simulink model "airgk"  (Simulink 3.00)
settings: Solver=ode45  StartTime=0  StopTime=Inf  RelTol=1e-3
libraries: simulink3 x21, airlib x1
(part 1 of 2)
settings Model: SaveTime=off  SaveOutput=off  RTWOptions="-aEnforceIntegerDowncast=1 -aFoldNonRolledExpr=1 -aInlineInvariantSignals=1 -aInlineParameters=0 -aLocalBlockOutputs=1 -aRollThreshold=5 -aZeroInternalMemoryAtStartup=1 -aZeroExternalMemoryAtStartup=1 -aInitFltsAndDblsToZero=1 -aGenerateReport=0 -aGenCodeOnly=0 -aRTWVerbose=1 -aIncludeHyperlinkInReport=0 -aLaunchReport=0 -aForceParamTrailComments=0 -aGenerateComments=1 -aIgnoreCustomStorageClasses=1 -aIncHierarchyInIds=0 -aMaxRTWIdLen=31 -aShowEliminatedStatements=0 -aPrefixModelToSubsysFcnNames=1 -aIncDataTypeInIds=0 -aInsertBlockDesc=0 -aSimulinkBlockComments=1 -aInlinedPrmAccess=\"Literals\"  -aSuppressErrorStatus=0 -aModelReferenceCompliant=1 -aSupportNonInlinedSFcns=1 -aSupportContinuousTime=1 -aSupportComplex=1 -aSupportNonFinite=1 -aSupportAbsoluteTime=1 -aTargetFcnLib=\"ansi_tfl_tmw.mat\" -aMultiInstanceERTCode=0 -aLogVarNameModifier=\"rt_\" -aIsPILTarget=0 -aCombineOutputUpdateFcns=0 -aGenerateASAP2=0 -aGenerateSampleERTMain=0 -aGenerateFullHeader=1 -aUtilityFuncGeneration=\"Auto\" -aIncludeFileDelimiter=\"Auto\" -aIncludeMdlTerminateFcn=1 -aPurelyIntegerCode=0 -aERTCustomFileBanners=0 -aRTWCAPIStates=0 -aRTWCAPIParams=0 -aRTWCAPISignals=0 -aMatFileLogging=1 -aGenFloatMathFcnCalls=\"ANSI_C\" -aExtModeMexFile=\"ext_comm\" -aExtModeTransport=0 -aExtModeStaticAllocSize=1000000 -aExtModeTesting=0 -aExtModeStaticAlloc=0 -aExtMode=0"  ExtModeTrigMode=normal  ExtModeArmWhenConnect=on  LastModifiedBy=gcampa

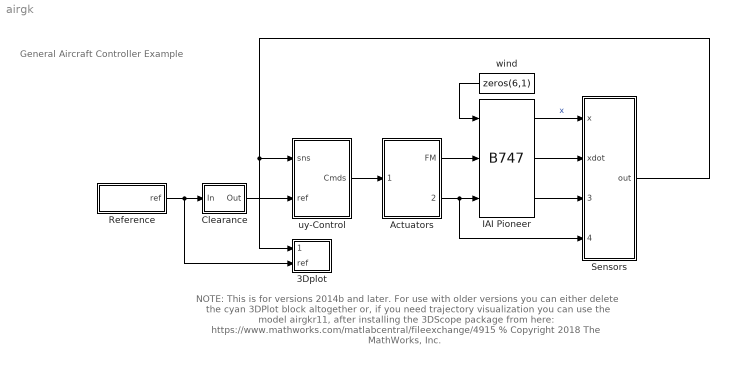
== system airgk ==
  note: General Aircraft
      | Controller Example
  note: NOTE: This is for versions 2014b and later. For use with older versions you can either delete the cyan 3DPlot block altogether or,
      | if you need trajectory visualization you can use the model airgkr11, after installing the 3DScope package from here:
      | https://www.mathworks.com/matlabcentral/fileexchange/4915                                             % Copyright 2018 The MathWorks, Inc.
  " IAI Pioneer " : airlib/B747  GM1="[0.5486  5.1511  2.8261   47.2259  90.9483  111.4754   0  -6.6462  0   190.512]"  CD_wind="[0.060  0.430  0  0.0180  0]"  CL_wind="[0.385  4.78  8.05  0.401  0]"  Cm_body="[0.194  -2.12   -36.6   -1.76    0]"  CY_body="[0   -0.819    0     0    0.191    0]"  Cl_body="[0   -0.023   -0.450   0.265   -0.161  -0.00229]"  Cn_body="[0    0.109  -0.110  -0.200    0.0200  -0.0917]"  x0="[60 -0.0293682 0   0 0 0   0 -0.0293682 0   0 0 60]"
  3Dplot : Subsystem
  Actuators : Subsystem
  Clearance : Subsystem  mask(Reference Position){FC=0, LC=0, HC=0}
      mask prompts: FC "Forward Clearance"; LC "Lateral Clearance"; HC "Altitude Clearance"
      mask help:
      | The input vector contains a position, velocity
      |   and two aditional signals. The output position
      |   is translated respect to the input of the quantities
      |   [FC, LC, HC] respectively behind, on the right
      |   and above the velocity vector direction.
      mask Help:
      | The input vector contains a position, velocity
      |   and two aditional signals. The output position
      |   is translated respect to the input of the quantities
      |   [FC, LC, HC] respectively behind, on the right
      |   and above the velocity vector direction.
  Reference : Subsystem  mask(Reference Path Generation){Px=[0          2000          2000             0             0             0], Py=[0             0          2000          2000          1000             0], Ph=[60           100            60           500            60            60], Pt=[0   33.3400   66.6800  100.8105  119.0191  135.6858], T=0.05}
      mask prompts: Px "X Positions"; Py "Y Positions"; Ph "H Positions"; Pt "Time"; T "Sample Time"
      mask help: This block generates a 3D trajectory. The output is a vector containing the position and velocity of a point that sequentially visits each X,Y,Z position at the corresponding time. The velocity is constant between one visited point and the next.
      mask Help: This block generates a 3D trajectory. The output is a vector containing the position and velocity of a point that sequentially visits each X,Y,Z position at the corresponding time. The velocity is constant between one visited point and the next.
  Sensors : Subsystem
  uy-Control : Subsystem  mask(General Nonlinear Aircraft Controller){GM1=[0.5486  5.1511  2.8261   47.2259  90.9483  111.4754   0  -6.6462  0   190.512], CD_wind=[0.060  0.430  0  0.0180  0], CL_wind=[0.385  4.78  8.05  0.401  0], Cm_body=[0.194  -2.12   -36.6   -1.76    0], Cl_body=[0   -0.023   -0.450   0.265   -0.161  -0.00229], Cn_body=[0    0.109  -0.110  -0.200    0.0200  -0.0917], K=[-6.75 9 -9 13.5 0.3], THor=15, Ts=0.05}
      mask prompts: GM1 "Geometry and Mass : [cbar   b    S    Ix   Iy   Iz   Jxy  Jxz  Jyz  m]"; CD_wind "Aerodynamic D-Force Derivatives : [CD0 CDa CDq CDde CDih]"; CL_wind "Aerodynamic L-Force Derivatives : [CL0 CLa CLq CLde CLih]"; Cm_body "Aerodynamic Y-Moment Derivatives : [Cm0 Cma Cmq Cmde Cmih]"; Cl_body "Aerodynamic X-moment Derivatives : [Cl0 Clb Clp Clr Clda Cldr]"; Cn_body "Aerodynamic Z-moment Derivatives : [Cn0 Cnb Cnp Cnr Cnda Cndr]"; K "Controller Coefficients: [Ka Kb Kc Kd Ku]"; THor "Horizon Time"; Ts "Sampling Time"
      mask help:
      | This block is a general feedback linearization controller for aircraft.
      | The first input is a vector contains the 12 aircraft states.
      | The second input contains the reference position and velocity.
      | The output contains the commanded deflections (elevator, aileron and rudder) and the thrust force along the body x axis. Geometry, Mass and Aerodynamic Derivatives should match the ones of the aircraft to be controlled. Ka,Kb,Kc,Kd, are the state space (scalar) coefficients of a PID controller for the feedback linearized attitude dynamics, which behaves as a double integrator system. Ku is the proportional forward velocity controller. The Horizon time is the approximated time lag between reference and actual trajectory. Usually only the aircraft related coefficients need to be changed when applying the controller to a different aircraft.
      mask Help:
      | <p>
      |   This block is a general feedback linearization controller for aircraft.
      |   The first input is a vector contains the 12 aircraft states.
      |   The second input contains the reference position and velocity.
      |   The output contains the commanded deflections (elevator,
      |   aileron and rudder) and the thrust force along the body x axis.
      |   Geometry, Mass and Aerodynamic Derivatives should match the
      |   ones of the aircraft to be controlled. Ka,Kb,Kc,Kd, are the state space
      |   (scalar) coefficients of a PID controller for the feedback linearized
      |   attitude dynamics, which behaves as a double integrator system.
      |   Ku is the proportional forward velocity controller. The Horizon time
      |   is the approximated time lag between reference and actual trajectory.
      |   Usually only the aircraft related coefficients need to be changed
      |   when applying the controller to a different aircraft.
      | </p>
      | <p>
      | Note that neither flaps nor stabilators can be used by this control. Also, this control can be used only when the linearized system having thrust, elevators, ailerons, rudder as inputs, and speed, roll, pitch, yaw as outputs is non-minimum phase. Usually such a system has 2 zeros on the negative real axis, related to alpha and beta respectively. Only occasionally the zero related to beta is on the positive real axis. In those cases the system is non-minimum phase and this controller is not usable anymore.
      | </p>
      | <p>
      | The control surface sign conventions are the same adopted in books such as Stevens-Lewis and Etkin, and in many flight simulators,
      | including the FDC toolbox. <br>
      | Specifically, positive elevator deflection causes negative pitching moment (Cmde &#60 0), positive rudder deflection causes negative yawing
      | moment (Cndr &#60 0), and positive aileron deflection causes negative rolling moment (Clda &#60 0). Another way to say the same thing is
      | that, the positive elevators deflection is Trailing Edge Down (TED), the positive rudder(s) deflection is Trailing Edge Left (TEL), and,
      | taking as TED the positive ailerons deflection, da=K*(da_right-da_left), with K usually equal to 1 (FDC) or 1/2.
      | </p>
      | <p>
      | Since this block is largely based on the FDC toolbox, i redirect you to the FDC Toolbox manual, for a good explanation of the underlying
      | components. Besides the mask and the fact that the aerodynamic derivatives are expressed in the stability axis, the only relevant difference
      | with the FDC toolbox is that in the computation of the aerodynamic forces, q is normalized as q*cbar/2V instead of q*cbar/V. The majority
      | of aeronautics books that i've seen use q*cbar/2V.
      | </p>
      | <p>
      | Please note that the International Measurement System is adopted. So, lengths are in meters, masses in Kg, and inertia moments in Kg*m^2.
      | Moreover, forces are in N, moments in N*m, accelerations in g, and angles in radians. For those that use the english system, here are some useful
      | conversion factors: <br>
      | 1 ft   = 0.3048 m, 1 lb   = 0.4536 Kg, 1 slug = 14.593903 Kg ,  1 slug*ft^2 = 1.355818 Kg*m^2
      | <br>
      | </p>
      | <p>
      | Finally, there is an <A HREF="http://www.aae.uiuc.edu/m-selig/apasim/Aircraft-uiuc.html">excellent source</A> of aircraft aerodynamic data
      | which is mantained by Michael S. Selig, Rob Deters, and Glen Dimock at the university of Urbana-Champaign. To use any of the given models
      | you just need to type the supplied aircraft data in the block mask.
      | </p>
      | <p>
      | <p>
      | July 2006, Giampiero Campa
      | </p>
      | </p>
      mask Display: disp('General\nAircraft\nController')
  wind : Constant  Orientation=left  Value=zeros(6,1)
  wires:
  Reference/1(ref) -> 3Dplot/2(ref), Clearance/1(In)
  " IAI Pioneer "/1 -> Sensors/1(x)  "x"
  wind/1 -> " IAI Pioneer "/1
  Actuators/1(FM) -> " IAI Pioneer "/2
  uy-Control/1(Cmds) -> Actuators/1(Cmds)
  Clearance/1(Out) -> uy-Control/2(ref)
  " IAI Pioneer "/2 -> Sensors/2(xdot)
  " IAI Pioneer "/3 -> Sensors/3(others)
  Actuators/2(Deltas) -> " IAI Pioneer "/3, Sensors/4(controls)
  Sensors/1(out) -> 3Dplot/1(meas), uy-Control/1(sns)

== system airgk/3Dplot ==
  note: Set Camera position to [0 0 1] for 2D view
  meas : Inport  Port=1  PortWidth=-1  SampleTime=-1  DataType=auto
      settings: SignalType=auto
  ref : Inport  Port=2  PortWidth=-1  SampleTime=-1  DataType=auto
      settings: SignalType=auto
  3D Graph : S-Function  LoadFcn=if exist('sfun3d','file'), sfun3d([],[],[],'LoadBlock'); end  FunctionName=sfun3d  Parameters=ax,T,np,cp,gd,ls,mk,mx,hd,tb  PortCounts=[]  SFunctionModules=''  mask(3D Graph){np=2, ax=[-1 3 -1 3 0 0.5]*1e3, mx=1e3, T=0.1, cp=[-10 -20 3]*1e3, gd=on, hd=on, tb=off, ls=-, mk=none}
      mask prompts: np "Number of moving points (lines)"; ax "Range: [xmin xmax  ymin ymax zmin zmax]"; mx "Max number of points in each line"; T "Sampling Time"; cp "Camera position (use [0 0 1] for 2D XY view)"; gd "Grid (on\"; hd "off)"; tb "HeadMarkers (on\"; ls "off)"; mk "Toolbar (on\"
      mask help:
      | This block plots the position of several points in the XYZ space. The input contains the coordinates of all the points (x1,y1,z1,x2,y2,z2,...).
      | The number of moving points (lines), the XYZ ranges, sampling time, camera position, and grid (among other things) can be set as mask parameters.
      settings: CopyFcn=if exist('sfun3d','file'), sfun3d([],[],[],'CopyBlock'); end  DeleteFcn=if exist('sfun3d','file'), sfun3d([],[],[],'DeleteBlock'); end  NameChangeFcn=if exist('sfun3d','file'), sfun3d([],[],[],'NameChange'); end
      mask Help:
      | This block plots the position of several points in the XYZ space. The input contains the coordinates of all the points (x1,y1,z1,x2,y2,z2,...).
      | The number of moving points (lines), the XYZ ranges, sampling time, camera position, and grid (among other things) can be set as mask parameters.
      mask StyleString: edit,edit,edit,edit,edit,checkbox,checkbox,checkbox,popup(-|--|:|-.|none),popup(none|.|+|o|*|x|square|diamond|v|^|>|<|pentagram|hexagram)
      mask Display: plot([.05 .95 .95 .05 .05],[.45 .45 .95 .95 .45], 0.5+cos(0:0.1:2*pi)*0.3,0.7+sin(0:0.1:2*pi)*0.2)
  Mux3 : Mux  Inputs=[3 3]
  real xyz : Selector  Elements=10:12  InputPortWidth=12
  ref xyz : Selector  Elements=1:3  InputPortWidth=6
  wires:
  real xyz/1 -> Mux3/1
  ref/1 -> ref xyz/1
  meas/1 -> real xyz/1
  ref xyz/1 -> Mux3/2
  Mux3/1 -> 3D Graph/1

== system airgk/Actuators ==
  Cmds : Inport  Port=1  PortWidth=-1  SampleTime=-1  DataType=auto
      settings: SignalType=auto
  Demux2 : Demux  Outputs=4
  Mux : Mux  Inputs=[1 1 1 1]
  Mux1 : Mux  Inputs=[1 5]
      settings: DisplayOption=none
  const : Constant  Value=zeros(5,1)
  FM : Outport  Port=1
  Deltas : Outport  Port=2
  wires:
  Mux/1 -> Deltas/1
  Mux1/1 -> FM/1
  const/1 -> Mux1/2
  Demux2/4 -> Mux/4, Mux1/1  "Insert Engine Model Here ( Transfer Function + Limiter + Rate Limiter)"
  Cmds/1 -> Demux2/1
  Demux2/3 -> Mux/3  "Insert Rudder Actuator Model Here ( Transfer Function + Limiter + Rate Limiter)"
  Demux2/2 -> Mux/2  "Insert Aileron Actuator Model Here ( Transfer Function + Limiter + Rate Limiter)"
  Demux2/1 -> Mux/1  "Insert Elevator Actuator Model Here ( Transfer Function + Limiter + Rate Limiter)"

== system airgk/Clearance ==
  In : Inport  Port=1  PortWidth=-1  SampleTime=-1  DataType=auto
      settings: SignalType=auto
  Mux2 : Mux  Inputs=[1 1 1 3]
  Sum1 : Sum  Inputs=|+-  SaturateOnIntegerOverflow=on
  const : Constant  Value=-HC
  r1 : Fcn  Expr=(u[5]*LC+u[4]*FC)/sqrt(u[4]^2+u[5]^2)
  r2 : Fcn  Expr=(-u[4]*LC+u[5]*FC)/sqrt(u[4]^2+u[5]^2)
  velocity : Constant  Value=[0 0 0]
  Out : Outport  Port=1
  wires:
  Sum1/1 -> Out/1
  Mux2/1 -> Sum1/2
  In/1 -> r2/1, r1/1, Sum1/1
  r1/1 -> Mux2/1
  r2/1 -> Mux2/2
  const/1 -> Mux2/3
  velocity/1 -> Mux2/4

== system airgk/Reference ==
  Clock : Clock
      settings: DisplayTime=off  Decimation=10
  Delay : UnitDelay  X0=[Px(1) Py(1) Ph(1)]  SampleTime=T
  Derivative : Subsystem  mask(Time Derivative){x0=[Px(1) Py(1) Ph(1)]'-[Px(2)-Px(1) Py(2)-Py(1) Ph(2)-Ph(1)]'/(Pt(2)-Pt(1))*T, T=T}
      mask prompts: x0 "Initial Condition"; T "Sampling Time"
      mask help:
      | First order approximation of the time derivative of the input signal,
      |   the original one is buggy.
  Hd(t) : Lookup  InputValues=Pt  OutputValues=Ph
  Horizon Time : Constant  Value=0
  Math Function : Math  Operator=mod  OutputSignalType=auto
  Mux : Mux  Inputs=3
  Mux2 : Mux  Inputs=[3 3]
  Sum2 : Sum  Inputs=++|  SaturateOnIntegerOverflow=on
  Time Limit : Constant  Value=Pt(end)
  Xd(t) : Lookup  InputValues=Pt  OutputValues=Px
  Yd(t) : Lookup  InputValues=Pt  OutputValues=Py
  ref : Outport  Port=1
  wires:
  Mux/1 -> Derivative/1(x), Delay/1
  Time Limit/1 -> Math Function/2
  Math Function/1 -> Hd(t)/1, Yd(t)/1, Xd(t)/1
  Clock/1 -> Sum2/2
  Horizon Time/1 -> Sum2/1
  Sum2/1 -> Math Function/1
  Hd(t)/1 -> Mux/3
  Yd(t)/1 -> Mux/2
  Xd(t)/1 -> Mux/1
  Delay/1 -> Mux2/1
  Derivative/1(xdot) -> Mux2/2
  Mux2/1 -> ref/1

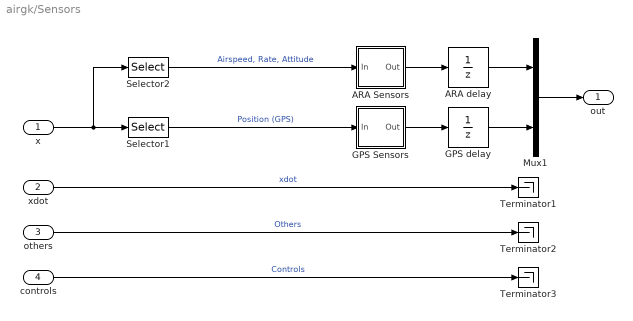
== system airgk/Sensors ==
  x : Inport  Port=1  PortWidth=-1  SampleTime=-1  DataType=auto
      settings: SignalType=auto
  xdot : Inport  Port=2  PortWidth=-1  SampleTime=-1  DataType=auto
      settings: SignalType=auto
  others : Inport  Port=3  PortWidth=-1  SampleTime=-1  DataType=auto
      settings: SignalType=auto
  controls : Inport  Port=4  PortWidth=-1  SampleTime=-1  DataType=auto
      settings: SignalType=auto
  ARA Sensors : Subsystem
  ARA delay : UnitDelay  X0="[60 -0.0293682 0   0 0 0   0 -0.0293682 0]"  SampleTime=0.05
  GPS Sensors : Subsystem
  GPS delay : UnitDelay  X0="[-2.5  0  60]"  SampleTime=0.05
  Mux1 : Mux  Inputs=[9 3]
  Selector1 : Selector  Elements=[10 11 12]  InputPortWidth=12
  Selector2 : Selector  Elements=[1:9]  InputPortWidth=12
  Terminator1 : Terminator
  Terminator2 : Terminator
  Terminator3 : Terminator
  out : Outport  Port=1
  wires:
  controls/1 -> Terminator3/1  "Controls"
  others/1 -> Terminator2/1  "Others"
  xdot/1 -> Terminator1/1  "xdot"
  Mux1/1 -> out/1
  GPS Sensors/1(Out) -> GPS delay/1
  GPS delay/1 -> Mux1/2
  ARA delay/1 -> Mux1/1
  Selector1/1 -> GPS Sensors/1(In)  "Position (GPS)"
  ARA Sensors/1(Out) -> ARA delay/1
  Selector2/1 -> ARA Sensors/1(In)  "Airspeed, Rate, Attitude"
  x/1 -> Selector2/1, Selector1/1

== system airgk/uy-Control ==
  sns : Inport  Port=1  PortWidth=-1  SampleTime=-1  DataType=auto
      settings: SignalType=auto
  ref : Inport  Port=2  PortWidth=-1  SampleTime=-1  DataType=auto
      settings: SignalType=auto
  4CmdsuKinInv : Subsystem  mask(Inverse Nonlinear Aircraft Model){Psi0=0, T=Ts}
      mask prompts: Psi0 "Initial Psi (used for Turn Coordination Derivative)"; T "Sampling Time (used for Turn Coordination Derivative)"
      mask help:
      | This block uses an exact turn coordination constraint
      |   to obtain velocity and attitude commands from desired accelerations.
      |   The first input contains the desired derivatives of the position (x,y,H).
      |   The second input contains the actual state of the aircraft.
      |   The first and second outputs contain respectively the commanded
      |   euler angles and the speed along the x axis (u=Vcos(a)cos(b)).
      |   NB : The International measurement system (MKS) is adopted.
      mask Help:
      | This block uses an exact turn coordination constraint
      |   to obtain velocity and attitude commands from desired accelerations.
      |   The first input contains the desired derivatives of the position (x,y,H).
      |   The second input contains the actual state of the aircraft.
      |   The first and second outputs contain respectively the commanded
      |   euler angles and the speed along the x axis (u=Vcos(a)cos(b)).
      |   NB : The International measurement system (MKS) is adopted.
      mask Display: disp('u-Inverse\nKinematic\nModel')
  Ku : Gain  Gain=K(5)  SaturateOnIntegerOverflow=on
  Selector1 : Selector  Elements=[9 8 7]  InputPortWidth=12
  State-Space : StateSpace  A=K(1)*eye(3)  B=K(2)*eye(3)  C=K(3)*eye(3)  D=K(4)*eye(3)  X0=0
  Sum1 : Sum  Inputs=|+-  SaturateOnIntegerOverflow=on
  Sum2 : Sum  Inputs=-+|  SaturateOnIntegerOverflow=on
  Vcmd Generator : Subsystem  mask(Velocity Command Generator){Kp=1, Kv=0, THor=THor, T=Ts}
      mask prompts: Kp "Position Error Gain"; Kv "Velocity Error Gain"; THor "Horizon Time"; T "Sample Time"
      mask help:
      | The first input is a reference position and velocity vector,
      |   the second one is a current position and velocity vector.
      |   The output is a filtered command in xyHdot .
      mask Help:
      | The first input is a reference position and velocity vector,
      |   the second one is a current position and velocity vector.
      |   The output is a filtered command in xyHdot .
  u : Fcn  Expr=u[1]*cos(u[2])*cos(u[3])
  uDynInv : Subsystem  mask(Inverse Nonlinear Aircraft Model){GM1=GM1, CD_wind=CD_wind, CL_wind=CL_wind, Cm_body=Cm_body, Cl_body=Cl_body, Cn_body=Cn_body}
      mask prompts: GM1 "Geometry, Mass : [cbar   b    S    Ix   Iy   Iz   Jxy  Jxz  Jyz  m]"; CD_wind "Aerodynamic D-Force Derivatives : [CD0 CDa CDq CDde CDih]"; CL_wind "Aerodynamic L-Force Derivatives : [CL0 CLa CLq CLde CLih]"; Cm_body "Aerodynamic Y-Moment Derivatives : [Cm0 Cma Cmq Cmde Cmih]"; Cl_body "Aerodynamic X-moment Derivatives : [Cl0 Clb Clp Clr Clda Cldr]"; Cn_body "Aerodynamic Z-moment Derivatives : [Cn0 Cnb Cnp Cnr Cnda Cndr]"
      mask help:
      | The first and second inputs contain the desired double derivatives
      |   of the attitude (roll, pitch, and yaw) and the desired detivative of
      |   u=V*cos(alpha)*cos(beta), which is the speed along the x body axis.
      |   The third input contains the actual state of the aircraft.
      |   The output contains the commanded deflections (elevator,
      |   aileron and rudder) and thrust force along the body x axis.
      |   NB : The International measurement system (MKS) is adopted.
      mask init:
      | AM=zeros(6,19);
      | AM(1,[1 2 9 11 12])=reshape(CD_wind,1,5);
      | AM(3,[1 2 9 11 12])=reshape(CL_wind,1,5);
      | AM(5,[1 2 9 11 12])=reshape(Cm_body,1,5);
      | AM(4,[1 5 8 10 13 14])=reshape(Cl_body,1,6);
      | AM(6,[1 5 8 10 13 14])=reshape(Cn_body,1,6);
      | 
      | Ix=GM1(4);Iy=GM1(5);Iz=GM1(6);
      | Jxy=GM1(7);Jxz=GM1(8);Jyz=GM1(9);
      | 
      | detI = Ix*Iy*Iz - 2*Jxy*Jxz*Jyz - Ix*Jyz^2 - Iy*Jxz^2 - Iz*Jxy^2;
      | I1   = Iy*Iz - Jyz^2;I2   = Jxy*Iz + Jyz*Jxz;
      | I3   = Jxy*Jyz + Iy*Jxz;I4   = Ix*Iz - Jxz^2;
      | I5   = Ix*Jyz + Jxy*Jxz;I6   = Ix*Iy - Jxy^2;
      | 
      | Pl  = I1/detI; Pm = I2/detI; Pn = I3/detI;
      | Ppp = -(Jxz*I2 - Jxy*I3)/detI;Ppq = (Jxz*I1 - Jyz*I2 - (Iy-Ix)*I3)/detI;
      | Ppr = -(Jxy*I1 + (Ix-Iz)*I2 - Jyz*I3)/detI;Pqq = (Jyz*I1 - Jxy*I3)/detI;
      | Pqr = -((Iz-Iy)*I1 - Jxy*I2 + Jxz*I3)/detI;Prr = -(Jyz*I1 - Jxz*I2)/detI;
      | 
      | Ql  = I2/detI; Qm = I4/detI; Qn = I5/detI;
      | Qpp = -(Jxz*I4 - Jxy*I5)/detI;Qpq = (Jxz*I2 - Jyz*I4 - (Iy-Ix)*I5)/detI;
      | Qpr = -(Jxy*I2 + (Ix-Iz)*I4 - Jyz*I5)/detI;Qqq = (Jyz*I2 - Jxy*I5)/detI;
      | Qqr = -((Iz-Iy)*I2 - Jxy*I4 + Jxz*I5)/detI;Qrr = -(Jyz*I2 - Jxz*I4)/detI;
      | 
      | Rl  = I3/detI; Rm = I5/detI; Rn = I6/detI;
      | Rpp = -(Jxz*I5 - Jxy*I6)/detI;
      | Rpq = (Jxz*I3 - Jyz*I5 - (Iy-Ix)*I6)/detI;
      | Rpr = -(Jxy*I3 + (Ix-Iz)*I5 - Jyz*I6)/detI;
      | Rqq = (Jyz*I3 - Jxy*I6)/detI;
      | Rqr = -((Iz-Iy)*I3 - Jxy*I5 + Jxz*I6)/detI;
      | Rrr = -(Jyz*I3 - Jxz*I5)/detI;
      | 
      | GM2 = [  Pl   Pm   Pn   Ppp  Ppq  Ppr  Pqq  Pqr  Prr ;
      |                Ql  Qm   Qn   Qpp  Qpq  Qpr  Qqq  Qqr  Qrr ;
      |                Rl  Rm   Rn   Rpp  Rpq  Rpr  Rqq  Rqr  Rrr ];
      | 
      | xfix=1;
      mask Help:
      | <p>
      | This block is an inverse nonlinear 6DOF aircraft model, with a very accurate built-in atmosphere model and constant aerodynamic derivatives.
      | The architecture of the block is largely based on the Aircraft block provided by the <A
      | HREF="http://www.mathworks.com/matlabcentral/fileexchange/loadFile.do?objectId=252&objectType=file">FDC toolbox</A> (Marc Rauw, 1993-2000).
      | </p>
      | <p>
      | The geometric and inertal data of the aircraft are entered as parameters in the first row of the mask, sampling time is the last parameter. The other rows contain the non-dimensional aerodynamic derivatives.
      | </p>
      | <p>
      |   The first and second inputs contain the desired double derivatives
      |   of the attitude (roll, pitch, and yaw) and the desired detivative of
      |   u=V*cos(alpha)*cos(beta), which is the speed along the x body axis.
      |   The third input contains the actual state of the aircraft.
      |   The output contains the commanded deflections (elevator,
      |   aileron and rudder) and thrust force along the body x axis.
      | </p>
      | <p>
      | Note that neither flaps nor stabilators can be used by this control.
      | </p>
      | <p>
      | The control surface sign conventions are the same adopted in books such as Stevens-Lewis and Etkin, and in many flight simulators,
      | including the FDC toolbox. <br>
      | Specifically, positive elevator deflection causes negative pitching moment (Cmde &#60 0), positive rudder deflection causes negative yawing
      | moment (Cndr &#60 0), and positive aileron deflection causes negative rolling moment (Clda &#60 0). Another way to say the same thing is
      | that, the positive elevators deflection is Trailing Edge Down (TED), the positive rudder(s) deflection is Trailing Edge Left (TEL), and,
      | taking as TED the positive ailerons deflection, da=K*(da_right-da_left), with K usually equal to 1 (FDC) or 1/2.
      | </p>
      | <p>
      | Since this block is largely based on the FDC toolbox, i redirect you to the FDC Toolbox manual, for a good explanation of the underlying
      | components. Besides the mask and the fact that the aerodynamic derivatives are expressed in the stability axis, the only relevant difference
      | with the FDC toolbox is that in the computation of the aerodynamic forces, q is normalized as q*cbar/2V instead of q*cbar/V. The majority
      | of aeronautics books that i've seen use q*cbar/2V.
      | </p>
      | <p>
      | Please note that the International Measurement System is adopted. So, lengths are in meters, masses in Kg, and inertia moments in Kg*m^2.
      | Moreover, forces are in N, moments in N*m, accelerations in g, and angles in radians. For those that still use the english system, here are some useful
      | conversion factors: <br>
      | 1 ft   = 0.3048 m, 1 lb   = 0.4536 Kg, 1 slug = 14.593903 Kg ,  1 slug*ft^2 = 1.355818 Kg*m^2
      | <br>
      | </p>
      | <p>
      | Finally, there is an <A HREF="http://www.aae.uiuc.edu/m-selig/apasim/Aircraft-uiuc.html">excellent source</A> of aircraft aerodynamic data
      | which is mantained by Michael S. Selig, Rob Deters, and Glen Dimock at the university of Urbana-Champaign. To use any of the given models
      | you just need to type the supplied aircraft data in the block mask.
      | </p>
      | <p>
      | <p>
      | Feb 2004, Giampiero Campa
      | </p>
      | </p>
      mask Display: disp('4 Cmds\nu-Inverse\nAircraft\nModel')
  Cmds : Outport  Port=1
  wires:
  ref/1 -> Vcmd Generator/1(ref)
  Vcmd Generator/1(xyHdot des) -> 4CmdsuKinInv/1(pdotdes)
  Sum2/1 -> State-Space/1
  Ku/1 -> uDynInv/2(udotdes)
  State-Space/1 -> uDynInv/1(ftpddotdes)
  sns/1 -> Selector1/1, 4CmdsuKinInv/2(x), Vcmd Generator/2(sns), u/1, uDynInv/3(x)
  Selector1/1 -> Sum2/1  "ftp"
  4CmdsuKinInv/1(rpycmd) -> Sum2/2  "rpy des"
  uDynInv/1(Cmds) -> Cmds/1
  4CmdsuKinInv/2(ucmd) -> Sum1/1  "u des"
  u/1 -> Sum1/2  "u"
  Sum1/1 -> Ku/1

== system airgk/Reference/Derivative ==
  x : Inport  Orientation=left  Port=1  PortWidth=-1  SampleTime=-1  DataType=auto
      settings: SignalType=auto
  Product2 : Product  Orientation=left  Inputs=/*  SaturateOnIntegerOverflow=on
  Sum4 : Sum  Orientation=left  Inputs=|+-  SaturateOnIntegerOverflow=on
  Unit Delay1 : UnitDelay  Orientation=left  X0=x0  SampleTime=T
  Zero-Order Hold1 : ZeroOrderHold  Orientation=left  SampleTime=T
  m : Constant  Orientation=left  Value=T
  xdot : Outport  Orientation=left  Port=1
  wires:
  Sum4/1 -> Product2/2
  Unit Delay1/1 -> Sum4/2
  Zero-Order Hold1/1 -> Sum4/1, Unit Delay1/1
  m/1 -> Product2/1
  Product2/1 -> xdot/1
  x/1 -> Zero-Order Hold1/1

== system airgk/Sensors/ARA Sensors ==
  note: Insert ARA (Airspeed, Rate, Attitude) Sensors Model Here
      | ( Transfer Functions + Limiters + Noise)
  In : Inport  Port=1  PortWidth=-1  SampleTime=-1  DataType=auto
      settings: SignalType=auto
  Demux : Demux  Outputs=9
  Mux1 : Mux  Inputs=9
  Out : Outport  Port=1
  wires:
  Demux/7 -> Mux1/7
  In/1 -> Demux/1
  Mux1/1 -> Out/1
  Demux/1 -> Mux1/1
  Demux/2 -> Mux1/2
  Demux/3 -> Mux1/3
  Demux/4 -> Mux1/4
  Demux/5 -> Mux1/5
  Demux/6 -> Mux1/6
  Demux/8 -> Mux1/8
  Demux/9 -> Mux1/9

== system airgk/Sensors/GPS Sensors ==
  note: Add GPS Noine Model Here
  In : Inport  Port=1  PortWidth=-1  SampleTime=-1  DataType=auto
      settings: SignalType=auto
  Out : Outport  Port=1
  wires:
  In/1 -> Out/1

== system airgk/uy-Control/4CmdsuKinInv ==
  pdotdes : Inport  Port=1  PortWidth=-1  SampleTime=-1  DataType=auto
      settings: SignalType=auto
  x : Inport  Port=2  PortWidth=-1  SampleTime=-1  DataType=auto
      settings: SignalType=auto
  Demux : Demux  Outputs=3
  Exact Turn Coordination : Subsystem
  Mux1 : Mux  Inputs=3
  Mux2 : Mux  Inputs=[3 12]
  a2c  xy : Subsystem  mask(Continuous Atan2 Function){L=4, T=T}
      mask prompts: L "Maximum angular distance covered during the sample time (< 2*pi)"; T "Sample Time"
      mask help:
      | This atan2 does not jump between pi and -pi.
      |   It is assumed that the inputs changes smoothly in time,
      |   specifically it is assumed that the maximum magnitude of the
      |   angular velocity of the input point [x,y] is less than L/T [rad/sec],
      |   where L and T are the first and second parameters in the mask.
  a2c xz : Subsystem  mask(Continuous Atan2 Function){L=4, T=T}
      mask prompts: L "Maximum angular distance covered during the sample time (< 2*pi)"; T "Sample Time"
      mask help:
      | This atan2 does not jump between pi and -pi.
      |   It is assumed that the inputs changes smoothly in time,
      |   specifically it is assumed that the maximum magnitude of the
      |   angular velocity of the input point [x,y] is less than L/T [rad/sec],
      |   where L and T are the first and second parameters in the mask.
  function : Fcn  Expr=sqrt(abs(u[1]^2+u[2]^2+u[3]^2))*cos(u[3+2])*cos(u[3+3])
  norm Vxy : Fcn  Expr=sqrt(u[1]^2+u[2]^2)
  rpycmd : Outport  Port=1
  ucmd : Outport  Port=2
  wires:
  x/1 -> Exact Turn Coordination/1(x), Mux2/2
  Exact Turn Coordination/3(psi) -> Mux1/3
  Mux1/1 -> rpycmd/1
  Exact Turn Coordination/2(theta) -> Mux1/2
  Exact Turn Coordination/1(phi) -> Mux1/1
  a2c  xy/1(a) -> Exact Turn Coordination/2(chi)  "chi"
  norm Vxy/1 -> a2c xz/2(x)
  Demux/3 -> a2c xz/1(y)
  Demux/2 -> a2c  xy/1(y)
  Demux/1 -> a2c  xy/2(x)
  a2c xz/1(a) -> Exact Turn Coordination/3(gamma)  "gamma"
  pdotdes/1 -> norm Vxy/1, Mux2/1, Demux/1  "xyHdotdes"
  function/1 -> ucmd/1
  Mux2/1 -> function/1

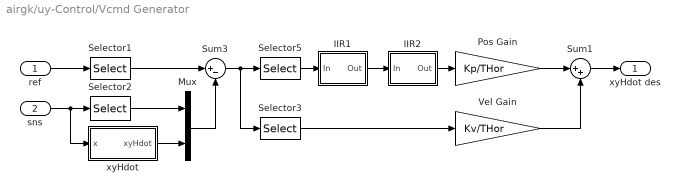
== system airgk/uy-Control/Vcmd Generator ==
  ref : Inport  Port=1  PortWidth=-1  SampleTime=-1  DataType=auto
      settings: SignalType=auto
  sns : Inport  Port=2  PortWidth=-1  SampleTime=-1  DataType=auto
      settings: SignalType=auto
  IIR1 : Subsystem  mask(Discrete Time Second Order IIR){ni=3, w=20/THor, x=1, x0=0, T=T}
      mask prompts: ni "Number of Channels"; w "Poles Magnitude (m)"; x "Poles Damping (x)"; x0 "Initial Condition"; T "Sample Time"
      mask help:
      | Each channel has the transfer function :
      |   1-2*cos(sqrt(1-x^2)*m*T)*exp(-x*m*T)+exp(-2*x*m*T) /
      |   1-2*cos(sqrt(1-x^2)*m*T)*exp(-x*m*T)z^-1+exp(-2*x*m*T)z^-2
      |   which is a good (pz-matched) approximation of
      |   m^2/(s^2+2xms+m^2) if 10*m*T<pi
      |   The initial condition is in discrete time for the whole system.
      mask init:
      | A=[];B=[];C=[];D=[];
      | for i=1:ni,
      | A=[A,zeros(size(A,1),2);zeros(2,size(A,2)),[0 1; -exp(-2*x*w*T) 2*cos(sqrt(1-x^2)*w*T)*exp(-x*w*T)]];
      | B=[B,zeros(size(B,1),1);zeros(2,size(B,2)),[0;1+exp(-2*x*w*T)-2*cos(sqrt(1-x^2)*w*T)*exp(-x*w*T)]];
      | C=[C,zeros(size(C,1),2);zeros(1,size(C,2)),[-exp(-2*x*w*T)  2*cos(sqrt(1-x^2)*w*T)*exp(-x*w*T)]];
      | D=[D,zeros(size(D,1),1);zeros(1,size(D,2)),1+exp(-2*x*w*T)-2*cos(sqrt(1-x^2)*w*T)*exp(-x*w*T)];
      | end
      mask Help:
      | <p>
      |   Each channel has the transfer function :
      |   1-2*cos(sqrt(1-x^2)*m*T)*exp(-x*m*T)+exp(-2*x*m*T) /
      |   1-2*cos(sqrt(1-x^2)*m*T)*exp(-x*m*T)z^-1+exp(-2*x*m*T)z^-2
      |   which is a good (pz-matched) approximation of
      |   m^2/(s^2+2xms+m^2) if 10*m*T<pi
      | </p>
      | <p>
      |   The initial condition is in discrete time for the whole system.
      |    If the input is an m-channel vector u, being u0 at time zero,
      |    then a suitable initial condition is : x0=ones(2,1)*reshape(u0,1,m)
      | </p>
      mask Display: dpoly(w^2, [1 2*x*w w^2],'s')
  IIR2 : Subsystem  mask(Discrete Time Second Order IIR){ni=3, w=20/THor, x=1, x0=0, T=T}
      mask prompts: ni "Number of Channels"; w "Poles Magnitude (m)"; x "Poles Damping (x)"; x0 "Initial Condition"; T "Sample Time"
      mask help:
      | Each channel has the transfer function :
      |   1-2*cos(sqrt(1-x^2)*m*T)*exp(-x*m*T)+exp(-2*x*m*T) /
      |   1-2*cos(sqrt(1-x^2)*m*T)*exp(-x*m*T)z^-1+exp(-2*x*m*T)z^-2
      |   which is a good (pz-matched) approximation of
      |   m^2/(s^2+2xms+m^2) if 10*m*T<pi
      |   The initial condition is in discrete time for the whole system.
      mask init: same as airgk/uy-Control/Vcmd Generator/IIR1
      mask Help:
      | <p>
      |   Each channel has the transfer function :
      |   1-2*cos(sqrt(1-x^2)*m*T)*exp(-x*m*T)+exp(-2*x*m*T) /
      |   1-2*cos(sqrt(1-x^2)*m*T)*exp(-x*m*T)z^-1+exp(-2*x*m*T)z^-2
      |   which is a good (pz-matched) approximation of
      |   m^2/(s^2+2xms+m^2) if 10*m*T<pi
      | </p>
      | <p>
      |   The initial condition is in discrete time for the whole system.
      |    If the input is an m-channel vector u, being u0 at time zero,
      |    then a suitable initial condition is : x0=ones(2,1)*reshape(u0,1,m)
      | </p>
      mask Display: dpoly(w^2, [1 2*x*w w^2],'s')
  Mux : Mux  Inputs=[3 3]
  Pos Gain : Gain  Gain=Kp/THor  SaturateOnIntegerOverflow=on
  Selector1 : Selector  Elements=1:6  InputPortWidth=6
  Selector2 : Selector  Elements=10:12  InputPortWidth=12
  Selector3 : Selector  Elements=4:6  InputPortWidth=6
  Selector5 : Selector  Elements=1:3  InputPortWidth=6
  Sum1 : Sum  Inputs=|++  SaturateOnIntegerOverflow=on
  Sum3 : Sum  Inputs=|+-  SaturateOnIntegerOverflow=on
  Vel Gain : Gain  Gain=Kv/THor  SaturateOnIntegerOverflow=on
  xyHdot : Subsystem
      mask Type: uvw
      mask Description:
      | Calculation of earth-axes velocities
      | xdot,ydot,Hdot
      mask Display: disp('Earth-axes\nvelocities')
  xyHdot des : Outport  Port=1
  wires:
  Pos Gain/1 -> Sum1/1
  Vel Gain/1 -> Sum1/2
  Selector3/1 -> Vel Gain/1
  Sum1/1 -> xyHdot des/1
  ref/1 -> Selector1/1
  sns/1 -> Selector2/1, xyHdot/1(x)
  Sum3/1 -> Selector3/1, Selector5/1
  Selector5/1 -> IIR1/1(In)
  IIR1/1(Out) -> IIR2/1(In)
  IIR2/1(Out) -> Pos Gain/1
  Selector1/1 -> Sum3/1
  Selector2/1 -> Mux/1
  xyHdot/1(xyHdot) -> Mux/2
  Mux/1 -> Sum3/2

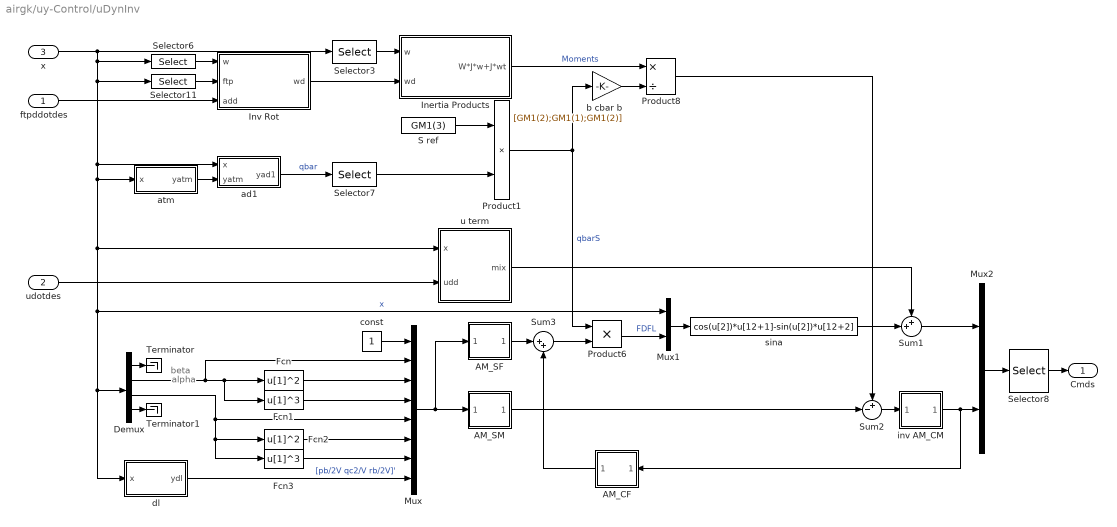
== system airgk/uy-Control/uDynInv ==
  note: beta
  note: alpha
  ftpddotdes : Inport  Port=1  PortWidth=-1  SampleTime=-1  DataType=auto
      settings: SignalType=auto
  udotdes : Inport  Port=2  PortWidth=-1  SampleTime=-1  DataType=auto
      settings: SignalType=auto
  x : Inport  Port=3  PortWidth=-1  SampleTime=-1  DataType=auto
      settings: SignalType=auto
  " u term" : Subsystem  mask(Vabdot){m=GM1(10)}
      mask prompts: m "Mass of the aircraft [kg]:"
      mask help: Calculation mixed aerodynamic forces
      mask Help: Calculation mixed aerodynamic forces
      mask Display: disp('Mixed\nAerodynamic\nForces')
  AM_CF : Subsystem  Orientation=left  mask(State Space){M=AM([1 3],[11 13 14])}
      mask prompts: M "Matrix"
      mask Display: disp('Matrix\nGain')
  AM_SF : Subsystem  mask(State Space){M=AM([1 3],1:10)}
      mask prompts: M "Matrix"
      mask Display: disp('Matrix\nGain')
  AM_SM : Subsystem  mask(State Space){M=AM(4:6,1:10)}
      mask prompts: M "Matrix"
      mask Display: disp('Matrix\nGain')
  Demux : Demux  Outputs=[1 1 1 9]
  Fcn : Fcn  Expr=u[1]^2
  Fcn1 : Fcn  Expr=u[1]^3
  Fcn2 : Fcn  Expr=u[1]^2
  Fcn3 : Fcn  Expr=u[1]^3
  Inertia Products : Subsystem
  Inv Rot : Subsystem
  Mux : Mux  Inputs=[1 1 1 1 1 1 1 3]
      settings: DisplayOption=none
  Mux1 : Mux  Inputs=[12 2]
      settings: DisplayOption=none
  Mux2 : Mux  Inputs=[1 3]
  Product1 : Product  Inputs=**  SaturateOnIntegerOverflow=on
  Product6 : Product  Inputs=**  SaturateOnIntegerOverflow=on
  Product8 : Product  Inputs=*/  SaturateOnIntegerOverflow=on
  S ref : Constant  Value=GM1(3)
  Selector11 : Selector  Elements=[9 8 7]  InputPortWidth=12
  Selector3 : Selector  Elements=[4 5 6]  InputPortWidth=12
  Selector6 : Selector  Elements=[4 5 6]  InputPortWidth=12
  Selector7 : Selector  Elements=3  InputPortWidth=3
  Selector8 : Selector  Elements=[2:4 1]  InputPortWidth=4
  Sum1 : Sum  Inputs=++|  SaturateOnIntegerOverflow=on
  Sum2 : Sum  Inputs=+-|  SaturateOnIntegerOverflow=on
  Sum3 : Sum  Inputs=|++  SaturateOnIntegerOverflow=on
  Terminator : Terminator
  Terminator1 : Terminator
  ad1 : Subsystem
      mask Type: Airdata1
      mask Description: Basic airdata variables
      mask Help: eval('fdchelp airdata1')
      mask Display: disp('Airdata1')
  atm : Subsystem
      mask Type: Atmosph
      mask Description: Atmosphere variables
      mask Help: eval('fdchelp atmosph')
      mask Display: disp('Atmosph')
  b cbar b : Gain  Gain=[GM1(2);GM1(1);GM1(2)]  SaturateOnIntegerOverflow=on
  const : Constant  Value=1
  dl : Subsystem  mask(Dimless){cbar=GM1(1), b=GM1(2)}
      mask prompts: cbar "Mean aerodynamic chord [m]:"; b "Wing span [m]:"
      mask help: Dimensionless rotational velocities.
      mask Help: eval('fdchelp dimless')
      mask Display: disp('Dimless')
  inv AM_CM : Subsystem  mask(State Space){M=pinv(AM(4:6,[11 13 14]))}
      mask prompts: M "Matrix"
      mask Display: disp('Matrix\nGain')
  sina : Fcn  Expr=cos(u[2])*u[12+1]-sin(u[2])*u[12+2]
  Cmds : Outport  Port=1
  wires:
  udotdes/1 -> " u term"/2(udd)
  " u term"/1(mix) -> Sum1/1
  Sum1/1 -> Mux2/1
  sina/1 -> Sum1/2
  Selector8/1 -> Cmds/1
  Mux1/1 -> sina/1
  Product6/1 -> Mux1/2  "FDFL"
  Sum3/1 -> Product6/2
  Sum2/1 -> inv AM_CM/1(In1)
  Inertia Products/1(W*J*w+J*wt) -> Product8/1  "Moments"
  Product1/1 -> b cbar b/1, Product6/1  "qbarS"
  b cbar b/1 -> Product8/2
  x/1 -> Selector11/1, " u term"/1(x), Mux1/1, Demux/1, dl/1(x), atm/1(x), ad1/1(x), Selector6/1, Selector3/1  "x"
  Demux/4 -> Terminator1/1
  Demux/1 -> Terminator/1
  const/1 -> Mux/1
  dl/1(ydl) -> Mux/8  "[pb/2V qc2/V rb/2V]'"
  Fcn2/1 -> Mux/6
  Demux/2 -> Fcn1/1, Fcn/1, Mux/2
  Demux/3 -> Fcn3/1, Fcn2/1, Mux/5
  Fcn3/1 -> Mux/7
  Fcn1/1 -> Mux/4
  Fcn/1 -> Mux/3
  Mux/1 -> AM_SM/1(In1), AM_SF/1(In1)
  AM_SM/1(Out1) -> Sum2/2
  AM_SF/1(Out1) -> Sum3/1
  AM_CF/1(Out1) -> Sum3/2
  inv AM_CM/1(Out1) -> AM_CF/1(In1), Mux2/2
  Product8/1 -> Sum2/1
  Mux2/1 -> Selector8/1
  atm/1(yatm) -> ad1/2(yatm)
  ftpddotdes/1 -> Inv Rot/3(add)
  Selector11/1 -> Inv Rot/2(ftp)
  Selector6/1 -> Inv Rot/1(w)
  Inv Rot/1(wd) -> Inertia Products/2(wd)
  S ref/1 -> Product1/1
  Selector3/1 -> Inertia Products/1(w)
  ad1/1(yad1) -> Selector7/1  "qbar"
  Selector7/1 -> Product1/2

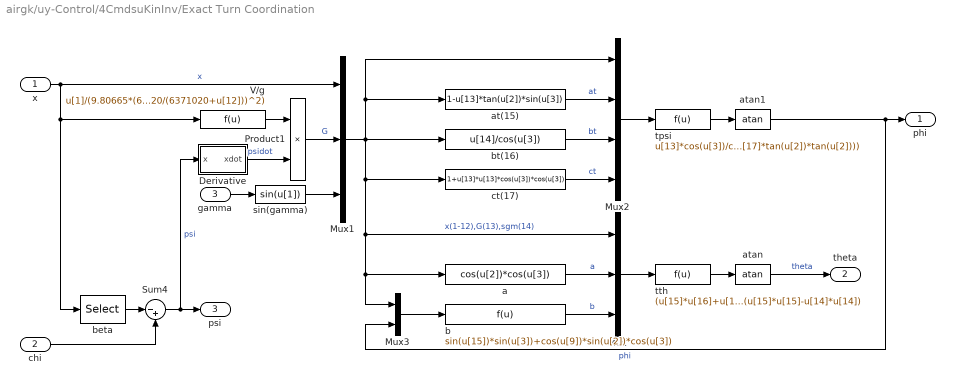
== system airgk/uy-Control/4CmdsuKinInv/Exact Turn Coordination ==
  x : Inport  Port=1  PortWidth=-1  SampleTime=-1  DataType=auto
      settings: SignalType=auto
  chi : Inport  Port=2  PortWidth=-1  SampleTime=-1  DataType=auto
      settings: SignalType=auto
  gamma : Inport  Port=3  PortWidth=-1  SampleTime=-1  DataType=auto
      settings: SignalType=auto
  Derivative : Subsystem  mask(Time Derivative){T=T, x0=Psi0}
      mask prompts: T "Sampling Time"; x0 "Initial Condition"
      mask help:
      | First order approximation of the time derivative of the input signal,
      |   the original one is buggy.
  Mux : Mux  Inputs=[14 1 1]
  Mux1 : Mux  Inputs=[12 1 1]
  Mux2 : Mux  Inputs=[14 1 1 1]
  Mux3 : Mux  Inputs=[14 1]
  Product1 : Product  Inputs=**  SaturateOnIntegerOverflow=on
  Sum4 : Sum  Inputs=|-+  SaturateOnIntegerOverflow=on
  V/g : Fcn  Expr=u[1]/(9.80665*(6371020/(6371020+u[12]))^2)
  a : Fcn  Expr=cos(u[2])*cos(u[3])
  at(15) : Fcn  Expr=1-u[13]*tan(u[2])*sin(u[3])
  atan : Trigonometry  Operator=atan  OutputSignalType=auto
  atan1 : Trigonometry  Operator=atan  OutputSignalType=auto
  b : Fcn  Expr=sin(u[15])*sin(u[3])+cos(u[9])*sin(u[2])*cos(u[3])
  beta : Selector  Elements=3  InputPortWidth=12
  bt(16) : Fcn  Expr=u[14]/cos(u[3])
  ct(17) : Fcn  Expr=1+u[13]*u[13]*cos(u[3])*cos(u[3])
  sin(gamma) : Fcn  Expr=sin(u[1])
  tpsi : Fcn  Expr=u[13]*cos(u[3])/cos(u[2])*(u[15]-u[16]*u[16]+u[16]*tan(u[2])*sqrt(abs(u[17]*(1-u[16]*u[16])+u[13]*u[13]*sin(u[3])*sin(u[3]))))/(u[15]*u[15]-u[16]*u[16]*(1+u[17]*tan(u[2])*tan(u[2])))
  tth : Fcn  Expr=(u[15]*u[16]+u[14]*sqrt(abs(u[15]*u[15]-u[14]*u[14]+u[16]*u[16])))/(u[15]*u[15]-u[14]*u[14])
  phi : Outport  Port=1
  theta : Outport  Port=2
  psi : Outport  Port=3
  wires:
  Sum4/1 -> Derivative/1(x), psi/1  "psi"
  beta/1 -> Sum4/1
  chi/1 -> Sum4/2
  Derivative/1(xdot) -> Product1/2  "psidot"
  V/g/1 -> Product1/1
  gamma/1 -> sin(gamma)/1
  sin(gamma)/1 -> Mux1/3
  Product1/1 -> Mux1/2  "G"
  Mux1/1 -> bt(16)/1, at(15)/1, Mux2/1, ct(17)/1, Mux/1, a/1, Mux3/1  "x(1-12),G(13),sgm(14)"
  Mux2/1 -> tpsi/1
  tth/1 -> atan/1
  Mux/1 -> tth/1
  Mux3/1 -> b/1
  a/1 -> Mux/2  "a"
  b/1 -> Mux/3  "b"
  atan1/1 -> Mux3/2, phi/1  "phi"
  tpsi/1 -> atan1/1
  at(15)/1 -> Mux2/2  "at"
  bt(16)/1 -> Mux2/3  "bt"
  ct(17)/1 -> Mux2/4  "ct"
  atan/1 -> theta/1  "theta"
  x/1 -> beta/1, V/g/1, Mux1/1  "x"

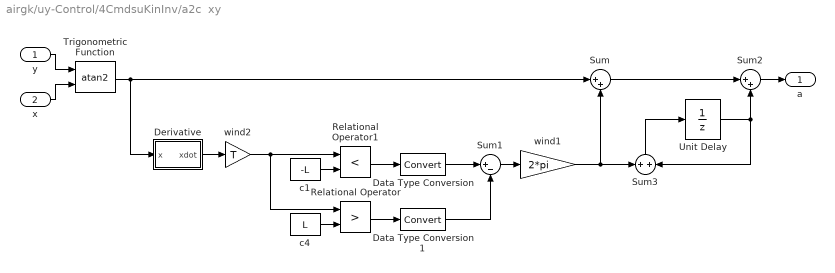
== system airgk/uy-Control/4CmdsuKinInv/a2c  xy ==
  y : Inport  Port=1  PortWidth=-1  SampleTime=-1  DataType=auto
      settings: SignalType=auto
  x : Inport  Port=2  PortWidth=-1  SampleTime=-1  DataType=auto
      settings: SignalType=auto
  Data Type Conversion : DataTypeConversion  DataType=double  SaturateOnIntegerOverflow=on
  Data Type Conversion1 : DataTypeConversion  DataType=double  SaturateOnIntegerOverflow=on
  Derivative : Subsystem  mask(Time Derivative){T=T}
      mask prompts: T "Sampling Time"
      mask help:
      | First order approximation of the time derivative of the input signal,
      |   the original one is buggy.
  Relational Operator : RelationalOperator  Operator=>
  Relational Operator1 : RelationalOperator  Operator=<
  Sum : Sum  Inputs=|++  SaturateOnIntegerOverflow=on
  Sum1 : Sum  Inputs=|+-  SaturateOnIntegerOverflow=on
  Sum2 : Sum  Inputs=|++  SaturateOnIntegerOverflow=on
  Sum3 : Sum  Orientation=up  Inputs=++  SaturateOnIntegerOverflow=on
  Trigonometric Function : Trigonometry  Operator=atan2  OutputSignalType=auto
  Unit Delay : UnitDelay  X0=0  SampleTime=T
  c1 : Constant  Value=-L
  c4 : Constant  Value=L
  wind1 : Gain  Gain=2*pi  SaturateOnIntegerOverflow=on
  wind2 : Gain  Gain=T  SaturateOnIntegerOverflow=on
  a : Outport  Port=1
  wires:
  Trigonometric Function/1 -> Sum/1, Derivative/1(x)
  Derivative/1(xdot) -> wind2/1
  wind2/1 -> Relational Operator/1, Relational Operator1/1
  c4/1 -> Relational Operator/2
  c1/1 -> Relational Operator1/2
  Relational Operator1/1 -> Data Type Conversion/1
  Relational Operator/1 -> Data Type Conversion1/1
  Data Type Conversion/1 -> Sum1/1
  Data Type Conversion1/1 -> Sum1/2
  Sum1/1 -> wind1/1
  wind1/1 -> Sum/2, Sum3/1
  Sum/1 -> Sum2/1
  Unit Delay/1 -> Sum2/2, Sum3/2
  Sum3/1 -> Unit Delay/1
  y/1 -> Trigonometric Function/1
  Sum2/1 -> a/1
  x/1 -> Trigonometric Function/2

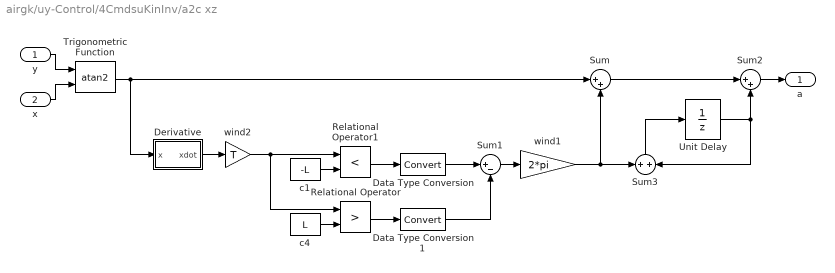
== system airgk/uy-Control/4CmdsuKinInv/a2c xz ==
  y : Inport  Port=1  PortWidth=-1  SampleTime=-1  DataType=auto
      settings: SignalType=auto
  x : Inport  Port=2  PortWidth=-1  SampleTime=-1  DataType=auto
      settings: SignalType=auto
  Data Type Conversion : DataTypeConversion  DataType=double  SaturateOnIntegerOverflow=on
  Data Type Conversion1 : DataTypeConversion  DataType=double  SaturateOnIntegerOverflow=on
  Derivative : Subsystem  mask(Time Derivative){T=T}
      mask prompts: T "Sampling Time"
      mask help:
      | First order approximation of the time derivative of the input signal,
      |   the original one is buggy.
  Relational Operator : RelationalOperator  Operator=>
  Relational Operator1 : RelationalOperator  Operator=<
  Sum : Sum  Inputs=|++  SaturateOnIntegerOverflow=on
  Sum1 : Sum  Inputs=|+-  SaturateOnIntegerOverflow=on
  Sum2 : Sum  Inputs=|++  SaturateOnIntegerOverflow=on
  Sum3 : Sum  Orientation=up  Inputs=++  SaturateOnIntegerOverflow=on
  Trigonometric Function : Trigonometry  Operator=atan2  OutputSignalType=auto
  Unit Delay : UnitDelay  X0=0  SampleTime=T
  c1 : Constant  Value=-L
  c4 : Constant  Value=L
  wind1 : Gain  Gain=2*pi  SaturateOnIntegerOverflow=on
  wind2 : Gain  Gain=T  SaturateOnIntegerOverflow=on
  a : Outport  Port=1
  wires:
  x/1 -> Trigonometric Function/2
  Sum2/1 -> a/1
  y/1 -> Trigonometric Function/1
  Sum3/1 -> Unit Delay/1
  Unit Delay/1 -> Sum3/2, Sum2/2
  Sum/1 -> Sum2/1
  wind1/1 -> Sum3/1, Sum/2
  Sum1/1 -> wind1/1
  Data Type Conversion1/1 -> Sum1/2
  Data Type Conversion/1 -> Sum1/1
  Relational Operator/1 -> Data Type Conversion1/1
  Relational Operator1/1 -> Data Type Conversion/1
  c1/1 -> Relational Operator1/2
  c4/1 -> Relational Operator/2
  wind2/1 -> Relational Operator1/1, Relational Operator/1
  Derivative/1(xdot) -> wind2/1
  Trigonometric Function/1 -> Derivative/1(x), Sum/1

== system airgk/uy-Control/Vcmd Generator/IIR1 ==
  In : Inport  Port=1  PortWidth=-1  SampleTime=-1  DataType=auto
      settings: SignalType=auto
  Discrete State-Space : DiscreteStateSpace  A=A  B=B  C=C  D=D  X0=x0  SampleTime=T
  Out : Outport  Port=1
  wires:
  In/1 -> Discrete State-Space/1
  Discrete State-Space/1 -> Out/1

== system airgk/uy-Control/Vcmd Generator/IIR2 ==
  In : Inport  Port=1  PortWidth=-1  SampleTime=-1  DataType=auto
      settings: SignalType=auto
  Discrete State-Space : DiscreteStateSpace  A=A  B=B  C=C  D=D  X0=x0  SampleTime=T
  Out : Outport  Port=1
  wires:
  In/1 -> Discrete State-Space/1
  Discrete State-Space/1 -> Out/1

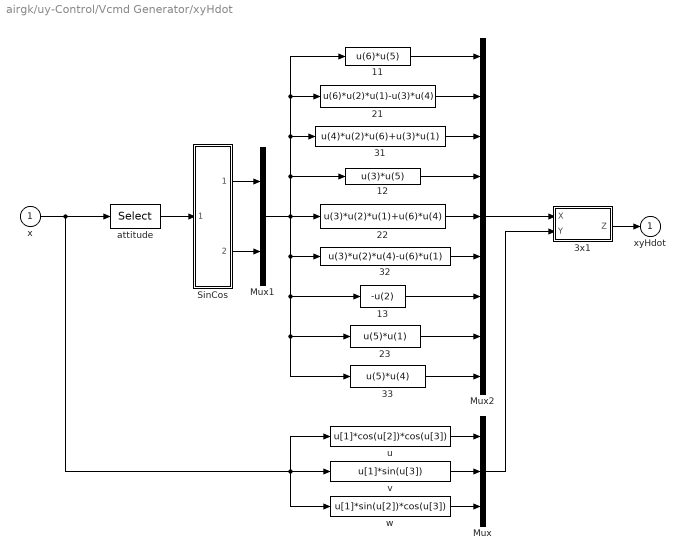
== system airgk/uy-Control/Vcmd Generator/xyHdot ==
  x : Inport  Port=1  PortWidth=-1  SampleTime=-1  DataType=auto
      settings: SignalType=auto
  11 : Fcn  Expr=u(6)*u(5)
  12 : Fcn  Expr=u(3)*u(5)
  13 : Fcn  Expr=-u(2)
  21 : Fcn  Expr=u(6)*u(2)*u(1)-u(3)*u(4)
  22 : Fcn  Expr=u(3)*u(2)*u(1)+u(6)*u(4)
  23 : Fcn  Expr=u(5)*u(1)
  31 : Fcn  Expr=u(4)*u(2)*u(6)+u(3)*u(1)
  32 : Fcn  Expr=u(3)*u(2)*u(4)-u(6)*u(1)
  33 : Fcn  Expr=u(5)*u(4)
  3x1 : Subsystem
      mask Type: 3x3 Matrix Multiplication
      mask Description:
      | Input 1   : elements of matrix X (3 by 3)
      |   Input 2   : elements of matrix Y (3 by 3)
      |   Output   : elements of matrix X*Y (3 by 3)
      mask Help:
      | <p>
      | Elements of input and output matrices are taken columnwise.
      | </p>
      mask Display: disp('Z=X*Y')
  Mux : Mux  Inputs=3
      settings: DisplayOption=none
  Mux1 : Mux  Inputs=2
  Mux2 : Mux  Inputs=9
  SinCos : Subsystem
      mask Type: SinCos
      mask Description: Compute the sine and cosine of input, u. u is in radians.
      mask Help: web(asbhelp);
      mask Display:
      | port_label('output',1,'sin(u)','texmode','on');
      | port_label('output',2,'cos(u)','texmode','on');
  attitude : Selector  Elements=[9 8 7]  InputPortWidth=12
  u : Fcn  Expr=u[1]*cos(u[2])*cos(u[3])
  v : Fcn  Expr=u[1]*sin(u[3])
  w : Fcn  Expr=u[1]*sin(u[2])*cos(u[3])
  xyHdot : Outport  Port=1
  wires:
  x/1 -> attitude/1, v/1, w/1, u/1
  33/1 -> Mux2/9
  23/1 -> Mux2/8
  13/1 -> Mux2/7
  32/1 -> Mux2/6
  22/1 -> Mux2/5
  12/1 -> Mux2/4
  31/1 -> Mux2/3
  21/1 -> Mux2/2
  11/1 -> Mux2/1
  SinCos/1(sin(theta)) -> Mux1/1
  SinCos/2(cos(theta)) -> Mux1/2
  Mux1/1 -> 22/1, 11/1, 21/1, 31/1, 12/1, 32/1, 13/1, 23/1, 33/1
  attitude/1 -> SinCos/1(theta)
  w/1 -> Mux/3
  u/1 -> Mux/1
  v/1 -> Mux/2
  Mux/1 -> 3x1/2(Y)
  Mux2/1 -> 3x1/1(X)
  3x1/1(Z) -> xyHdot/1

== system airgk/uy-Control/uDynInv/ u term ==
  x : Inport  Port=1  PortWidth=-1  SampleTime=-1  DataType=auto
      settings: SignalType=auto
  udd : Inport  Port=2  PortWidth=-1  SampleTime=-1  DataType=auto
      settings: SignalType=auto
  Mux1 : Mux  Inputs=[12 3 1]
  Term 1 with T=0 : Fcn  Expr=m*u[12+4]+m*(9.80665*(6371020/(6371020+u[12]))^2)*sin(u[8])+m*(u[5]*u[12+3]-u[6]*u[12+2])
  uvw : Subsystem
      mask Type: uvw
      mask Description:
      | Calculation of body-axes velocities
      | u, v, and w
      mask Help: eval('fdchelp uvw')
      mask Display: disp('Body-axes\nvelocities')
  mix : Outport  Port=1
  wires:
  x/1 -> Mux1/1, uvw/1(x)
  Mux1/1 -> Term 1 with T=0/1
  Term 1 with T=0/1 -> mix/1
  uvw/1(ybvel) -> Mux1/2
  udd/1 -> Mux1/3

== system airgk/uy-Control/uDynInv/AM_CF ==
  In1 : Inport  Port=1  PortWidth=-1  SampleTime=-1  DataType=auto
      settings: SignalType=auto
  Matrix Gain : StateSpace  A=[]  B=[]  C=[]  D=M  X0=0
  Out1 : Outport  Port=1
  wires:
  In1/1 -> Matrix Gain/1
  Matrix Gain/1 -> Out1/1

== system airgk/uy-Control/uDynInv/AM_SF ==
  In1 : Inport  Port=1  PortWidth=-1  SampleTime=-1  DataType=auto
      settings: SignalType=auto
  Matrix Gain : StateSpace  A=[]  B=[]  C=[]  D=M  X0=0
  Out1 : Outport  Port=1
  wires:
  In1/1 -> Matrix Gain/1
  Matrix Gain/1 -> Out1/1

== system airgk/uy-Control/uDynInv/AM_SM ==
  In1 : Inport  Port=1  PortWidth=-1  SampleTime=-1  DataType=auto
      settings: SignalType=auto
  Matrix Gain : StateSpace  A=[]  B=[]  C=[]  D=M  X0=0
  Out1 : Outport  Port=1
  wires:
  Matrix Gain/1 -> Out1/1
  In1/1 -> Matrix Gain/1
